simulink model "pfb_fir_real_plan"  (Simulink 7.6)
settings: Solver=ode45  StartTime=0.0  StopTime=10.0  RelTol=1e-3
undefined symbols (not defined in the file or in its folder): pfb_coeff_gen_calc_custom
libraries: xbsIndex_r4 x422, xbsReplacements_r4 x20, monroe_library x15
(part 1 of 4)
settings Model: Creator=monroe  LastModifiedBy=monroe

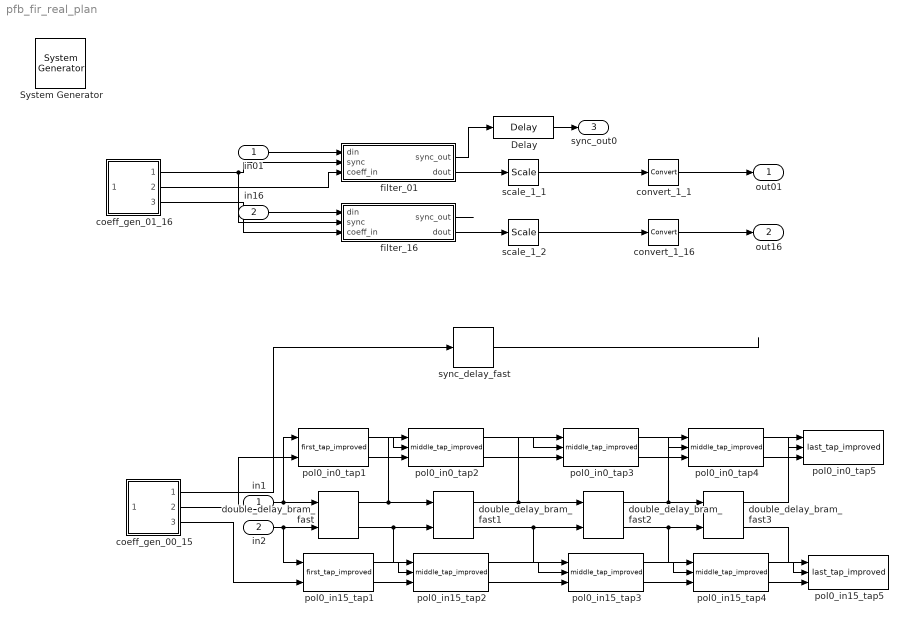
== system pfb_fir_real_plan ==
  in01 : Inport
  in16 : Inport  Port=2
  " System Generator" : xbsIndex_r4/ System Generator  Tag=genX  SystemSampleTime=-1  xilinxfamily=Virtex6  part=xc6vsx315t  speed=-3  package=ff1156  synthesis_tool=XST  clock_wrapper=Clock Enables  directory=./netlist  testbench=off  simulink_period=1  sysclk_period=10  dcm_input_clock_period=10  incr_netlist=off  trim_vbits=Everywhere in SubSystem  dbl_ovrd=According to Block Masks  core_generation=According to Block Masks  run_coregen=off  deprecated_control=off  eval_field=0  block_type=sysgen
  Delay : xbsIndex_r4/Delay  en=off  latency=1  dbl_ovrd=off  reg_retiming=off  block_type=delay
      settings: block_version=11.4
  coeff_gen_00_15 : Subsystem
      settings: AttributesFormatString=PFBSize=14, n_inputs=4, taps=2
  coeff_gen_01_16 : Subsystem
      settings: AttributesFormatString=PFBSize=14, n_inputs=4, taps=2
  convert_1_1 : xbsIndex_r4/Convert  arith_type="Signed  (2's comp)"  n_bits=18  bin_pt=17  quantization=Truncate  overflow=Wrap  en=off  latency=1  dbl_ovrd=off  pipeline=on  block_type=convert
      settings: block_version=11.4
  convert_1_16 : xbsIndex_r4/Convert  arith_type="Signed  (2's comp)"  n_bits=18  bin_pt=17  quantization=Truncate  overflow=Wrap  en=off  latency=1  dbl_ovrd=off  pipeline=on  block_type=convert
      settings: block_version=11.4
  double_delay_bram_fast{,1..3} (4 alike) : monroe_library/double_delay_bram_fast  SystemSampleTime=-1  delay_len=1024  bram_latency=3
  filter_01 : Subsystem
  filter_16 : Subsystem
  in1 : InportShadow  Port=1
  in2 : InportShadow  Port=2
  pol0_in0_tap1 : monroe_library/first_tap_improved  SystemSampleTime=-1  din_bit_width=18  din_bin_pt=17  coeff_bit_width=18  coeff_bin_pt=17
  pol0_in0_tap2 : monroe_library/middle_tap_improved  SystemSampleTime=-1  din_bit_width=18  din_bin_pt=17  coeff_bit_width=18  coeff_bin_pt=17  stage_num=2
  pol0_in0_tap3 : monroe_library/middle_tap_improved  SystemSampleTime=-1  din_bit_width=18  din_bin_pt=17  coeff_bit_width=18  coeff_bin_pt=17  stage_num=2
  pol0_in0_tap4 : monroe_library/middle_tap_improved  SystemSampleTime=-1  din_bit_width=18  din_bin_pt=17  coeff_bit_width=18  coeff_bin_pt=17  stage_num=2
  pol0_in0_tap5 : monroe_library/last_tap_improved  SystemSampleTime=-1  data_bin_pt=17  coeff_bin_pt=17  stage_num=6
  pol0_in15_tap1 : monroe_library/first_tap_improved  SystemSampleTime=-1  din_bit_width=18  din_bin_pt=17  coeff_bit_width=18  coeff_bin_pt=17
  pol0_in15_tap2 : monroe_library/middle_tap_improved  SystemSampleTime=-1  din_bit_width=18  din_bin_pt=17  coeff_bit_width=18  coeff_bin_pt=17  stage_num=2
  pol0_in15_tap3 : monroe_library/middle_tap_improved  SystemSampleTime=-1  din_bit_width=18  din_bin_pt=17  coeff_bit_width=18  coeff_bin_pt=17  stage_num=2
  pol0_in15_tap4 : monroe_library/middle_tap_improved  SystemSampleTime=-1  din_bit_width=18  din_bin_pt=17  coeff_bit_width=18  coeff_bin_pt=17  stage_num=2
  pol0_in15_tap5 : monroe_library/last_tap_improved  SystemSampleTime=-1  data_bin_pt=17  coeff_bin_pt=17  stage_num=6
  scale_1_1 : xbsIndex_r4/Scale  scale_factor=-1  dbl_ovrd=off  block_type=scale
  scale_1_2 : xbsIndex_r4/Scale  scale_factor=-1  dbl_ovrd=off  block_type=scale
  sync_delay_fast : monroe_library/sync_delay_fast  SystemSampleTime=-1  delay_len=1024*5+6+3-1
  out01 : Outport
  out16 : Outport  Port=2
  sync_out0 : Outport  Port=3
  wires:
  filter_16/1(sync_out) -> ?
  filter_16/2(dout) -> scale_1_2/1
  convert_1_16/1 -> out16/1
  scale_1_2/1 -> convert_1_16/1
  filter_01/2(dout) -> scale_1_1/1
  filter_01/1(sync_out) -> Delay/1
  Delay/1 -> sync_out0/1
  convert_1_1/1 -> out01/1
  scale_1_1/1 -> convert_1_1/1
  coeff_gen_01_16/1(sync_out) -> filter_01/2(sync), filter_16/2(sync)
  coeff_gen_01_16/3(coeff_rev) -> filter_16/3(coeff_in)
  coeff_gen_01_16/2(coeff) -> filter_01/3(coeff_in)
  in01/1 -> filter_01/1(din)
  in16/1 -> filter_16/1(din)
  in2/1 -> double_delay_bram_fast/2, pol0_in15_tap1/1
  in1/1 -> double_delay_bram_fast/1, pol0_in0_tap1/1
  double_delay_bram_fast/1 -> double_delay_bram_fast1/1, pol0_in0_tap2/1
  double_delay_bram_fast/2 -> double_delay_bram_fast1/2, pol0_in15_tap2/1
  double_delay_bram_fast1/1 -> double_delay_bram_fast2/1, pol0_in0_tap3/1
  double_delay_bram_fast1/2 -> double_delay_bram_fast2/2, pol0_in15_tap3/1
  double_delay_bram_fast2/1 -> double_delay_bram_fast3/1, pol0_in0_tap4/1
  double_delay_bram_fast2/2 -> double_delay_bram_fast3/2, pol0_in15_tap4/1
  double_delay_bram_fast3/1 -> pol0_in0_tap5/1
  double_delay_bram_fast3/2 -> pol0_in15_tap5/1
  coeff_gen_00_15/1(sync_out) -> sync_delay_fast/1
  sync_delay_fast/1 -> ?
  coeff_gen_00_15/2(coeff) -> pol0_in0_tap1/2
  coeff_gen_00_15/3(coeff_rev) -> pol0_in15_tap1/2
  pol0_in0_tap1/1 -> pol0_in0_tap2/2
  pol0_in0_tap1/2 -> pol0_in0_tap2/3
  pol0_in0_tap2/1 -> pol0_in0_tap3/2
  pol0_in0_tap2/2 -> pol0_in0_tap3/3
  pol0_in0_tap3/1 -> pol0_in0_tap4/2
  pol0_in0_tap3/2 -> pol0_in0_tap4/3
  pol0_in0_tap4/1 -> pol0_in0_tap5/2
  pol0_in0_tap4/2 -> pol0_in0_tap5/3
  pol0_in15_tap1/1 -> pol0_in15_tap2/2
  pol0_in15_tap1/2 -> pol0_in15_tap2/3
  pol0_in15_tap2/1 -> pol0_in15_tap3/2
  pol0_in15_tap2/2 -> pol0_in15_tap3/3
  pol0_in15_tap3/1 -> pol0_in15_tap4/2
  pol0_in15_tap3/2 -> pol0_in15_tap4/3
  pol0_in15_tap4/1 -> pol0_in15_tap5/2
  pol0_in15_tap4/2 -> pol0_in15_tap5/3

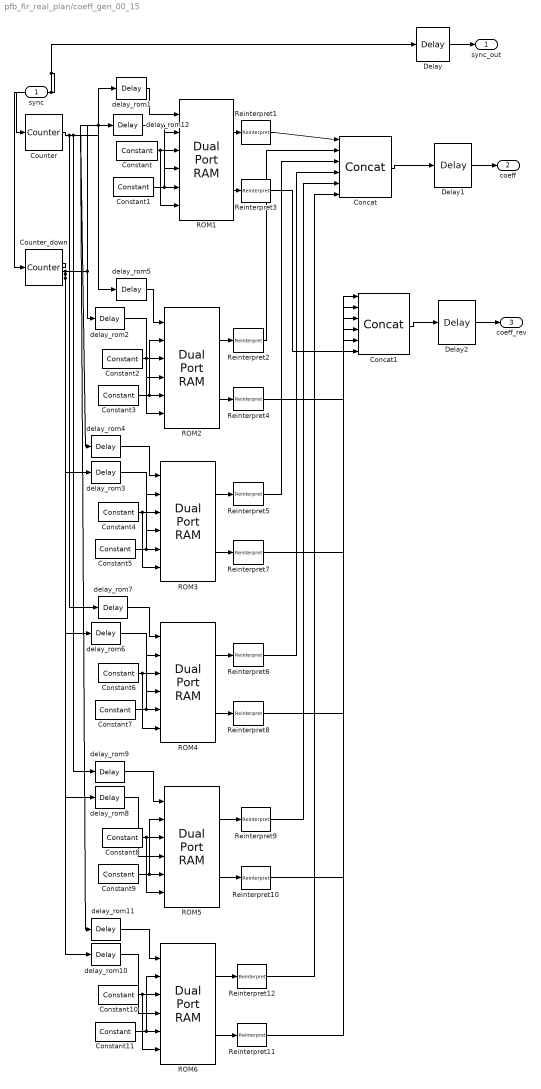
== system pfb_fir_real_plan/coeff_gen_00_15 ==
  sync : Inport
  Concat : xbsIndex_r4/Concat  num_inputs=6  dbl_ovrd=off  block_type=concat
      settings: block_version=9.1.01
  Concat1 : xbsIndex_r4/Concat  num_inputs=6  dbl_ovrd=off  block_type=concat
      settings: block_version=9.1.01
  Constant{,2,4,6,8,10} (6 alike) : xbsIndex_r4/Constant  arith_type=Boolean  const=0  n_bits=16  bin_pt=14  explicit_period=off  period=1  equ=P=C  opselect=C  inp2=PCIN>>17  opr=+  inp1=P  carry=CIN  dbl_ovrd=off  block_type=constant
  Constant{1,3,5,7,9,11} (6 alike) : xbsIndex_r4/Constant  arith_type=Signed (2's comp)  const=0  n_bits=18  bin_pt=17  explicit_period=off  period=1  equ=P=C  opselect=C  inp2=PCIN>>17  opr=+  inp1=P  carry=CIN  dbl_ovrd=off  block_type=constant
  Counter : xbsIndex_r4/Counter  cnt_type=Free Running  cnt_to=Inf  operation=Up  start_count=0  cnt_by_val=1  arith_type=Unsigned  n_bits=10  bin_pt=0  load_pin=off  rst=on  en=off  explicit_period=on  period=1  dbl_ovrd=off  use_behavioral_HDL=off  implementation=Fabric  use_rpm=on  block_type=counter
      settings: xl_area=[0, 0, 0, 0, 0, 0, 0]  block_version=9.1.01
  Counter_down : xbsIndex_r4/Counter  cnt_type=Free Running  cnt_to=Inf  operation=Up  start_count=2^10-1  cnt_by_val=-1  arith_type=Unsigned  n_bits=10  bin_pt=0  load_pin=off  rst=on  en=off  explicit_period=on  period=1  dbl_ovrd=off  use_behavioral_HDL=off  implementation=Fabric  use_rpm=on  block_type=counter
      settings: xl_area=[0, 0, 0, 0, 0, 0, 0]  block_version=9.1.01
  Delay : xbsIndex_r4/Delay  en=off  latency=4  dbl_ovrd=off  reg_retiming=off  block_type=delay
      settings: xl_area=[0, 0, 0, 0, 0, 0, 0]  block_version=9.1.01
  Delay1 : xbsIndex_r4/Delay  en=off  latency=1  dbl_ovrd=off  reg_retiming=off  block_type=delay
  Delay2 : xbsIndex_r4/Delay  en=off  latency=1  dbl_ovrd=off  reg_retiming=off  block_type=delay
  ROM1 : xbsIndex_r4/Dual Port RAM  depth=1024  initVector=pfb_coeff_gen_calc_custom(14,6,4,0,1,1)  distributed_mem=Block RAM  init_a=0  init_b=0  rst_a=off  rst_b=off  en_a=off  en_b=off  latency=3  write_mode_A=No Read On Write  write_mode_B=No Read On Write  dbl_ovrd=off  optimize=Area  use_rpm=on  block_type=dpram
  ROM2 : xbsIndex_r4/Dual Port RAM  depth=1024  initVector=pfb_coeff_gen_calc_custom(14,6,4,0,1,2)  distributed_mem=Block RAM  init_a=0  init_b=0  rst_a=off  rst_b=off  en_a=off  en_b=off  latency=3  write_mode_A=No Read On Write  write_mode_B=No Read On Write  dbl_ovrd=off  optimize=Area  use_rpm=on  block_type=dpram
  ROM3 : xbsIndex_r4/Dual Port RAM  depth=1024  initVector=pfb_coeff_gen_calc_custom(14,6,4,0,1,3)  distributed_mem=Block RAM  init_a=0  init_b=0  rst_a=off  rst_b=off  en_a=off  en_b=off  latency=3  write_mode_A=No Read On Write  write_mode_B=No Read On Write  dbl_ovrd=off  optimize=Area  use_rpm=on  block_type=dpram
  ROM4 : xbsIndex_r4/Dual Port RAM  depth=1024  initVector=pfb_coeff_gen_calc_custom(14,6,4,0,1,4)  distributed_mem=Block RAM  init_a=0  init_b=0  rst_a=off  rst_b=off  en_a=off  en_b=off  latency=3  write_mode_A=No Read On Write  write_mode_B=No Read On Write  dbl_ovrd=off  optimize=Area  use_rpm=on  block_type=dpram
  ROM5 : xbsIndex_r4/Dual Port RAM  depth=1024  initVector=pfb_coeff_gen_calc_custom(14,6,4,0,1,5)  distributed_mem=Block RAM  init_a=0  init_b=0  rst_a=off  rst_b=off  en_a=off  en_b=off  latency=3  write_mode_A=No Read On Write  write_mode_B=No Read On Write  dbl_ovrd=off  optimize=Area  use_rpm=on  block_type=dpram
  ROM6 : xbsIndex_r4/Dual Port RAM  depth=1024  initVector=pfb_coeff_gen_calc_custom(14,6,4,0,1,6)  distributed_mem=Block RAM  init_a=0  init_b=0  rst_a=off  rst_b=off  en_a=off  en_b=off  latency=3  write_mode_A=No Read On Write  write_mode_B=No Read On Write  dbl_ovrd=off  optimize=Area  use_rpm=on  block_type=dpram
  Reinterpret{1..12} (12 alike) : xbsIndex_r4/Reinterpret  force_arith_type=on  arith_type=Unsigned  force_bin_pt=on  bin_pt=0  block_type=reinterpret
      settings: infoedit="Changes signal type without altering the binary representation.   You can changed the signal between signed and unsigned, and relocate the binary point.<P><P>Hardware notes: In hardware this block costs nothing.<P><P>Example:  Suppose the input is 6 bits wide, signed, with 2 fractional bits, and the output is forced to unsigned with 0 fractional bits.  Then an input of -2.0 (1110.00 in binary 2's complement) becomes an output of 56 (111000 in binary)."  block_version=9.1.01
  delay_rom1 : xbsIndex_r4/Delay  en=off  latency=5  dbl_ovrd=off  reg_retiming=off  block_type=delay
  delay_rom10 : xbsIndex_r4/Delay  en=off  latency=5  dbl_ovrd=off  reg_retiming=off  block_type=delay
  delay_rom11 : xbsIndex_r4/Delay  en=off  latency=0  dbl_ovrd=off  reg_retiming=off  block_type=delay
  delay_rom12 : xbsIndex_r4/Delay  en=off  latency=0  dbl_ovrd=off  reg_retiming=off  block_type=delay
  delay_rom2 : xbsIndex_r4/Delay  en=off  latency=1  dbl_ovrd=off  reg_retiming=off  block_type=delay
  delay_rom3 : xbsIndex_r4/Delay  en=off  latency=2  dbl_ovrd=off  reg_retiming=off  block_type=delay
  delay_rom4 : xbsIndex_r4/Delay  en=off  latency=3  dbl_ovrd=off  reg_retiming=off  block_type=delay
  delay_rom5 : xbsIndex_r4/Delay  en=off  latency=4  dbl_ovrd=off  reg_retiming=off  block_type=delay
  delay_rom6 : xbsIndex_r4/Delay  en=off  latency=3  dbl_ovrd=off  reg_retiming=off  block_type=delay
  delay_rom7 : xbsIndex_r4/Delay  en=off  latency=2  dbl_ovrd=off  reg_retiming=off  block_type=delay
  delay_rom8 : xbsIndex_r4/Delay  en=off  latency=4  dbl_ovrd=off  reg_retiming=off  block_type=delay
  delay_rom9 : xbsIndex_r4/Delay  en=off  latency=1  dbl_ovrd=off  reg_retiming=off  block_type=delay
  sync_out : Outport
  coeff : Outport  Port=2
  coeff_rev : Outport  Port=3
  wires:
  Concat1/1 -> Delay2/1
  Delay2/1 -> coeff_rev/1
  Counter_down/1 -> delay_rom2/1, delay_rom12/1, delay_rom3/1, delay_rom6/1, delay_rom8/1, delay_rom10/1
  ROM1/2 -> Reinterpret3/1
  ROM2/1 -> Reinterpret2/1
  Constant3/1 -> ROM2/5, ROM2/2
  Constant2/1 -> ROM2/3, ROM2/6
  Constant1/1 -> ROM1/2, ROM1/5
  Constant/1 -> ROM1/6, ROM1/3
  Reinterpret2/1 -> Concat/2
  Reinterpret1/1 -> Concat/1
  ROM1/1 -> Reinterpret1/1
  Counter/1 -> delay_rom7/1, delay_rom1/1, delay_rom5/1, delay_rom4/1, delay_rom11/1, delay_rom9/1
  Delay1/1 -> coeff/1
  Concat/1 -> Delay1/1
  Delay/1 -> sync_out/1
  sync/1 -> Counter_down/1, Delay/1, Counter/1
  ROM2/2 -> Reinterpret4/1
  delay_rom1/1 -> ROM1/1
  delay_rom2/1 -> ROM2/4
  Constant5/1 -> ROM3/2, ROM3/5
  Constant4/1 -> ROM3/6, ROM3/3
  delay_rom3/1 -> ROM3/4
  delay_rom5/1 -> ROM2/1
  delay_rom4/1 -> ROM3/1
  Constant7/1 -> ROM4/5, ROM4/2
  Constant6/1 -> ROM4/3, ROM4/6
  delay_rom6/1 -> ROM4/4
  delay_rom7/1 -> ROM4/1
  Constant9/1 -> ROM5/2, ROM5/5
  Constant8/1 -> ROM5/6, ROM5/3
  delay_rom8/1 -> ROM5/4
  delay_rom9/1 -> ROM5/1
  Constant11/1 -> ROM6/5, ROM6/2
  Constant10/1 -> ROM6/3, ROM6/6
  delay_rom10/1 -> ROM6/4
  delay_rom11/1 -> ROM6/1
  Reinterpret3/1 -> Concat1/6
  Reinterpret4/1 -> Concat1/5
  ROM3/1 -> Reinterpret5/1
  ROM3/2 -> Reinterpret7/1
  ROM4/1 -> Reinterpret6/1
  ROM4/2 -> Reinterpret8/1
  ROM5/1 -> Reinterpret9/1
  ROM5/2 -> Reinterpret10/1
  ROM6/1 -> Reinterpret12/1
  ROM6/2 -> Reinterpret11/1
  Reinterpret5/1 -> Concat/3
  Reinterpret6/1 -> Concat/4
  Reinterpret9/1 -> Concat/5
  Reinterpret12/1 -> Concat/6
  Reinterpret7/1 -> Concat1/4
  Reinterpret8/1 -> Concat1/3
  Reinterpret10/1 -> Concat1/2
  Reinterpret11/1 -> Concat1/1
  delay_rom12/1 -> ROM1/4

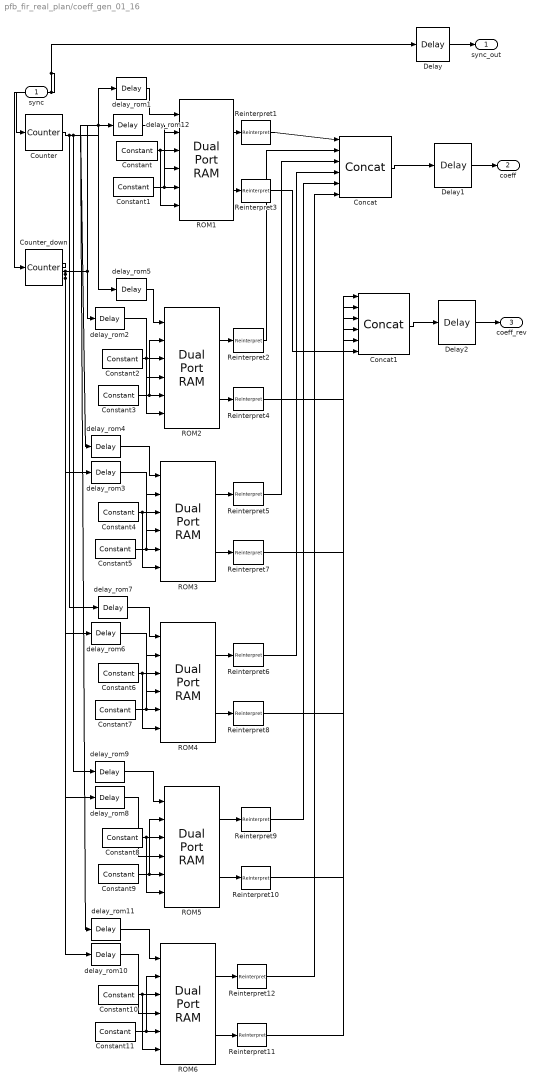
== system pfb_fir_real_plan/coeff_gen_01_16 ==
  sync : Inport
  Concat : xbsIndex_r4/Concat  num_inputs=6  dbl_ovrd=off  block_type=concat
      settings: block_version=9.1.01
  Concat1 : xbsIndex_r4/Concat  num_inputs=6  dbl_ovrd=off  block_type=concat
      settings: block_version=9.1.01
  Constant{,2,4,6,8,10} (6 alike) : xbsIndex_r4/Constant  arith_type=Boolean  const=0  n_bits=16  bin_pt=14  explicit_period=off  period=1  equ=P=C  opselect=C  inp2=PCIN>>17  opr=+  inp1=P  carry=CIN  dbl_ovrd=off  block_type=constant
  Constant{1,3,5,7,9,11} (6 alike) : xbsIndex_r4/Constant  arith_type=Signed (2's comp)  const=0  n_bits=18  bin_pt=17  explicit_period=off  period=1  equ=P=C  opselect=C  inp2=PCIN>>17  opr=+  inp1=P  carry=CIN  dbl_ovrd=off  block_type=constant
  Counter : xbsIndex_r4/Counter  cnt_type=Free Running  cnt_to=Inf  operation=Up  start_count=0  cnt_by_val=1  arith_type=Unsigned  n_bits=10  bin_pt=0  load_pin=off  rst=on  en=off  explicit_period=on  period=1  dbl_ovrd=off  use_behavioral_HDL=off  implementation=Fabric  use_rpm=on  block_type=counter
      settings: xl_area=[0, 0, 0, 0, 0, 0, 0]  block_version=9.1.01
  Counter_down : xbsIndex_r4/Counter  cnt_type=Free Running  cnt_to=Inf  operation=Up  start_count=2^10-1  cnt_by_val=-1  arith_type=Unsigned  n_bits=10  bin_pt=0  load_pin=off  rst=on  en=off  explicit_period=on  period=1  dbl_ovrd=off  use_behavioral_HDL=off  implementation=Fabric  use_rpm=on  block_type=counter
      settings: xl_area=[0, 0, 0, 0, 0, 0, 0]  block_version=9.1.01
  Delay : xbsIndex_r4/Delay  en=off  latency=4  dbl_ovrd=off  reg_retiming=off  block_type=delay
      settings: xl_area=[0, 0, 0, 0, 0, 0, 0]  block_version=9.1.01
  Delay1 : xbsIndex_r4/Delay  en=off  latency=1  dbl_ovrd=off  reg_retiming=off  block_type=delay
  Delay2 : xbsIndex_r4/Delay  en=off  latency=1  dbl_ovrd=off  reg_retiming=off  block_type=delay
  ROM1 : xbsIndex_r4/Dual Port RAM  depth=1024  initVector=pfb_coeff_gen_calc_custom(14,6,4,0,1,1)  distributed_mem=Block RAM  init_a=0  init_b=0  rst_a=off  rst_b=off  en_a=off  en_b=off  latency=3  write_mode_A=No Read On Write  write_mode_B=No Read On Write  dbl_ovrd=off  optimize=Area  use_rpm=on  block_type=dpram
  ROM2 : xbsIndex_r4/Dual Port RAM  depth=1024  initVector=pfb_coeff_gen_calc_custom(14,6,4,0,1,2)  distributed_mem=Block RAM  init_a=0  init_b=0  rst_a=off  rst_b=off  en_a=off  en_b=off  latency=3  write_mode_A=No Read On Write  write_mode_B=No Read On Write  dbl_ovrd=off  optimize=Area  use_rpm=on  block_type=dpram
  ROM3 : xbsIndex_r4/Dual Port RAM  depth=1024  initVector=pfb_coeff_gen_calc_custom(14,6,4,0,1,3)  distributed_mem=Block RAM  init_a=0  init_b=0  rst_a=off  rst_b=off  en_a=off  en_b=off  latency=3  write_mode_A=No Read On Write  write_mode_B=No Read On Write  dbl_ovrd=off  optimize=Area  use_rpm=on  block_type=dpram
  ROM4 : xbsIndex_r4/Dual Port RAM  depth=1024  initVector=pfb_coeff_gen_calc_custom(14,6,4,0,1,4)  distributed_mem=Block RAM  init_a=0  init_b=0  rst_a=off  rst_b=off  en_a=off  en_b=off  latency=3  write_mode_A=No Read On Write  write_mode_B=No Read On Write  dbl_ovrd=off  optimize=Area  use_rpm=on  block_type=dpram
  ROM5 : xbsIndex_r4/Dual Port RAM  depth=1024  initVector=pfb_coeff_gen_calc_custom(14,6,4,0,1,5)  distributed_mem=Block RAM  init_a=0  init_b=0  rst_a=off  rst_b=off  en_a=off  en_b=off  latency=3  write_mode_A=No Read On Write  write_mode_B=No Read On Write  dbl_ovrd=off  optimize=Area  use_rpm=on  block_type=dpram
  ROM6 : xbsIndex_r4/Dual Port RAM  depth=1024  initVector=pfb_coeff_gen_calc_custom(14,6,4,0,1,6)  distributed_mem=Block RAM  init_a=0  init_b=0  rst_a=off  rst_b=off  en_a=off  en_b=off  latency=3  write_mode_A=No Read On Write  write_mode_B=No Read On Write  dbl_ovrd=off  optimize=Area  use_rpm=on  block_type=dpram
  Reinterpret{1..12} (12 alike) : xbsIndex_r4/Reinterpret  force_arith_type=on  arith_type=Unsigned  force_bin_pt=on  bin_pt=0  block_type=reinterpret
      settings: infoedit="Changes signal type without altering the binary representation.   You can changed the signal between signed and unsigned, and relocate the binary point.<P><P>Hardware notes: In hardware this block costs nothing.<P><P>Example:  Suppose the input is 6 bits wide, signed, with 2 fractional bits, and the output is forced to unsigned with 0 fractional bits.  Then an input of -2.0 (1110.00 in binary 2's complement) becomes an output of 56 (111000 in binary)."  block_version=9.1.01
  delay_rom1 : xbsIndex_r4/Delay  en=off  latency=5  dbl_ovrd=off  reg_retiming=off  block_type=delay
  delay_rom10 : xbsIndex_r4/Delay  en=off  latency=5  dbl_ovrd=off  reg_retiming=off  block_type=delay
  delay_rom11 : xbsIndex_r4/Delay  en=off  latency=0  dbl_ovrd=off  reg_retiming=off  block_type=delay
  delay_rom12 : xbsIndex_r4/Delay  en=off  latency=0  dbl_ovrd=off  reg_retiming=off  block_type=delay
  delay_rom2 : xbsIndex_r4/Delay  en=off  latency=1  dbl_ovrd=off  reg_retiming=off  block_type=delay
  delay_rom3 : xbsIndex_r4/Delay  en=off  latency=2  dbl_ovrd=off  reg_retiming=off  block_type=delay
  delay_rom4 : xbsIndex_r4/Delay  en=off  latency=3  dbl_ovrd=off  reg_retiming=off  block_type=delay
  delay_rom5 : xbsIndex_r4/Delay  en=off  latency=4  dbl_ovrd=off  reg_retiming=off  block_type=delay
  delay_rom6 : xbsIndex_r4/Delay  en=off  latency=3  dbl_ovrd=off  reg_retiming=off  block_type=delay
  delay_rom7 : xbsIndex_r4/Delay  en=off  latency=2  dbl_ovrd=off  reg_retiming=off  block_type=delay
  delay_rom8 : xbsIndex_r4/Delay  en=off  latency=4  dbl_ovrd=off  reg_retiming=off  block_type=delay
  delay_rom9 : xbsIndex_r4/Delay  en=off  latency=1  dbl_ovrd=off  reg_retiming=off  block_type=delay
  sync_out : Outport
  coeff : Outport  Port=2
  coeff_rev : Outport  Port=3
  wires:
  delay_rom12/1 -> ROM1/4
  Reinterpret11/1 -> Concat1/1
  Reinterpret10/1 -> Concat1/2
  Reinterpret8/1 -> Concat1/3
  Reinterpret7/1 -> Concat1/4
  Reinterpret12/1 -> Concat/6
  Reinterpret9/1 -> Concat/5
  Reinterpret6/1 -> Concat/4
  Reinterpret5/1 -> Concat/3
  ROM6/2 -> Reinterpret11/1
  ROM6/1 -> Reinterpret12/1
  ROM5/2 -> Reinterpret10/1
  ROM5/1 -> Reinterpret9/1
  ROM4/2 -> Reinterpret8/1
  ROM4/1 -> Reinterpret6/1
  ROM3/2 -> Reinterpret7/1
  ROM3/1 -> Reinterpret5/1
  Reinterpret4/1 -> Concat1/5
  Reinterpret3/1 -> Concat1/6
  delay_rom11/1 -> ROM6/1
  delay_rom10/1 -> ROM6/4
  Constant10/1 -> ROM6/6, ROM6/3
  Constant11/1 -> ROM6/2, ROM6/5
  delay_rom9/1 -> ROM5/1
  delay_rom8/1 -> ROM5/4
  Constant8/1 -> ROM5/3, ROM5/6
  Constant9/1 -> ROM5/5, ROM5/2
  delay_rom7/1 -> ROM4/1
  delay_rom6/1 -> ROM4/4
  Constant6/1 -> ROM4/6, ROM4/3
  Constant7/1 -> ROM4/2, ROM4/5
  delay_rom4/1 -> ROM3/1
  delay_rom5/1 -> ROM2/1
  delay_rom3/1 -> ROM3/4
  Constant4/1 -> ROM3/3, ROM3/6
  Constant5/1 -> ROM3/5, ROM3/2
  delay_rom2/1 -> ROM2/4
  delay_rom1/1 -> ROM1/1
  ROM2/2 -> Reinterpret4/1
  sync/1 -> Counter/1, Delay/1, Counter_down/1
  Delay/1 -> sync_out/1
  Concat/1 -> Delay1/1
  Delay1/1 -> coeff/1
  Counter/1 -> delay_rom9/1, delay_rom11/1, delay_rom4/1, delay_rom5/1, delay_rom1/1, delay_rom7/1
  ROM1/1 -> Reinterpret1/1
  Reinterpret1/1 -> Concat/1
  Reinterpret2/1 -> Concat/2
  Constant/1 -> ROM1/3, ROM1/6
  Constant1/1 -> ROM1/5, ROM1/2
  Constant2/1 -> ROM2/6, ROM2/3
  Constant3/1 -> ROM2/2, ROM2/5
  ROM2/1 -> Reinterpret2/1
  ROM1/2 -> Reinterpret3/1
  Counter_down/1 -> delay_rom10/1, delay_rom8/1, delay_rom6/1, delay_rom3/1, delay_rom12/1, delay_rom2/1
  Delay2/1 -> coeff_rev/1
  Concat1/1 -> Delay2/1

== system pfb_fir_real_plan/filter_01 ==
  din : Inport
  sync : Inport  Port=2
  coeff_in : Inport  Port=3
  Delay1 : xbsIndex_r4/Delay  en=off  latency=1  dbl_ovrd=off  reg_retiming=off  block_type=delay
      settings: xl_area=[0, 0, 0, 0, 0, 0, 0]  block_version=9.1.01
  Reinterpret2 : xbsIndex_r4/Reinterpret  force_arith_type=on  arith_type="Signed  (2's comp)"  force_bin_pt=on  bin_pt=34  block_type=reinterpret
      settings: infoedit="Changes signal type without altering the binary representation.   You can changed the signal between signed and unsigned, and relocate the binary point.<br><br>Hardware notes: In hardware this block costs nothing.<br><br>Example:  Suppose the input is 6 bits wide, signed, with 2 fractional bits, and the output is forced to unsigned with 0 fractional bits.  Then an input of -2.0 (1110.00 in binary 2's complement) becomes an output of 56 (111000 in binary)."  block_version=11.3
  tap1 : Subsystem  AncestorBlock=casper_library/PFBs/tap_real
  tap2 : Subsystem  AncestorBlock=casper_library/PFBs/tap_real
  tap3 : Subsystem  AncestorBlock=casper_library/PFBs/tap_real
  tap4 : Subsystem  AncestorBlock=casper_library/PFBs/tap_real
  tap5 : Subsystem  AncestorBlock=casper_library/PFBs/tap_real
  tap6 : Subsystem  AncestorBlock=casper_library/PFBs/last_tap_real
  sync_out : Outport
  dout : Outport  Port=2
  wires:
  tap5/1(dout) -> tap6/1(din)
  tap5/2(sync_out) -> tap6/2(sync)
  tap5/3(coeff_out) -> tap6/3(coeff)
  tap5/4(taps_out) -> tap6/4(tap_in)
  tap1/1(dout) -> tap2/1(din)
  tap1/2(sync_out) -> tap2/2(sync)
  tap1/3(coeff_out) -> tap2/3(coeff)
  tap1/4(taps_out) -> tap2/4(tap_in)
  tap2/1(dout) -> tap3/1(din)
  tap2/2(sync_out) -> tap3/2(sync)
  tap2/3(coeff_out) -> tap3/3(coeff)
  tap2/4(taps_out) -> tap3/4(tap_in)
  tap3/1(dout) -> tap4/1(din)
  tap3/2(sync_out) -> tap4/2(sync)
  tap3/3(coeff_out) -> tap4/3(coeff)
  tap3/4(taps_out) -> tap4/4(tap_in)
  tap4/1(dout) -> tap5/1(din)
  tap4/2(sync_out) -> tap5/2(sync)
  tap4/3(coeff_out) -> tap5/3(coeff)
  tap4/4(taps_out) -> tap5/4(tap_in)
  tap6/2(tap_out) -> Reinterpret2/1
  Delay1/1 -> tap1/1(din)
  din/1 -> Delay1/1
  tap6/1(sync_out) -> sync_out/1
  sync/1 -> tap1/2(sync)
  Reinterpret2/1 -> dout/1
  coeff_in/1 -> tap1/3(coeff)

== system pfb_fir_real_plan/filter_16 ==
  din : Inport
  sync : Inport  Port=2
  coeff_in : Inport  Port=3
  Delay1 : xbsIndex_r4/Delay  en=off  latency=1  dbl_ovrd=off  reg_retiming=off  block_type=delay
      settings: xl_area=[0, 0, 0, 0, 0, 0, 0]  block_version=9.1.01
  Reinterpret2 : xbsIndex_r4/Reinterpret  force_arith_type=on  arith_type="Signed  (2's comp)"  force_bin_pt=on  bin_pt=34  block_type=reinterpret
      settings: infoedit="Changes signal type without altering the binary representation.   You can changed the signal between signed and unsigned, and relocate the binary point.<br><br>Hardware notes: In hardware this block costs nothing.<br><br>Example:  Suppose the input is 6 bits wide, signed, with 2 fractional bits, and the output is forced to unsigned with 0 fractional bits.  Then an input of -2.0 (1110.00 in binary 2's complement) becomes an output of 56 (111000 in binary)."  block_version=11.3
  tap1 : Subsystem  AncestorBlock=casper_library/PFBs/tap_real
  tap2 : Subsystem  AncestorBlock=casper_library/PFBs/tap_real
  tap3 : Subsystem  AncestorBlock=casper_library/PFBs/tap_real
  tap4 : Subsystem  AncestorBlock=casper_library/PFBs/tap_real
  tap5 : Subsystem  AncestorBlock=casper_library/PFBs/tap_real
  tap6 : Subsystem  AncestorBlock=casper_library/PFBs/last_tap_real
  sync_out : Outport
  dout : Outport  Port=2
  wires:
  coeff_in/1 -> tap1/3(coeff)
  Reinterpret2/1 -> dout/1
  sync/1 -> tap1/2(sync)
  tap6/1(sync_out) -> sync_out/1
  din/1 -> Delay1/1
  Delay1/1 -> tap1/1(din)
  tap6/2(tap_out) -> Reinterpret2/1
  tap4/4(taps_out) -> tap5/4(tap_in)
  tap4/3(coeff_out) -> tap5/3(coeff)
  tap4/2(sync_out) -> tap5/2(sync)
  tap4/1(dout) -> tap5/1(din)
  tap3/4(taps_out) -> tap4/4(tap_in)
  tap3/3(coeff_out) -> tap4/3(coeff)
  tap3/2(sync_out) -> tap4/2(sync)
  tap3/1(dout) -> tap4/1(din)
  tap2/4(taps_out) -> tap3/4(tap_in)
  tap2/3(coeff_out) -> tap3/3(coeff)
  tap2/2(sync_out) -> tap3/2(sync)
  tap2/1(dout) -> tap3/1(din)
  tap1/4(taps_out) -> tap2/4(tap_in)
  tap1/3(coeff_out) -> tap2/3(coeff)
  tap1/2(sync_out) -> tap2/2(sync)
  tap1/1(dout) -> tap2/1(din)
  tap5/4(taps_out) -> tap6/4(tap_in)
  tap5/3(coeff_out) -> tap6/3(coeff)
  tap5/2(sync_out) -> tap6/2(sync)
  tap5/1(dout) -> tap6/1(din)

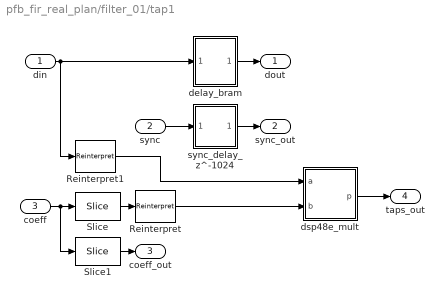
== system pfb_fir_real_plan/filter_01/tap1 ==
  din : Inport
  sync : Inport  Port=2
  coeff : Inport  Port=3
  Reinterpret : xbsIndex_r4/Reinterpret  force_arith_type=on  arith_type="Signed  (2's comp)"  force_bin_pt=on  bin_pt=17  block_type=reinterpret
      settings: infoedit="Changes signal type without altering the binary representation.   You can changed the signal between signed and unsigned, and relocate the binary point.<br><br>Hardware notes: In hardware this block costs nothing.<br><br>Example:  Suppose the input is 6 bits wide, signed, with 2 fractional bits, and the output is forced to unsigned with 0 fractional bits.  Then an input of -2.0 (1110.00 in binary 2's complement) becomes an output of 56 (111000 in binary)."  block_version=9.1.01
  Reinterpret1 : xbsIndex_r4/Reinterpret  force_arith_type=on  arith_type="Signed  (2's comp)"  force_bin_pt=on  bin_pt=17  block_type=reinterpret
      settings: infoedit="Changes signal type without altering the binary representation.   You can changed the signal between signed and unsigned, and relocate the binary point.<br><br>Hardware notes: In hardware this block costs nothing.<br><br>Example:  Suppose the input is 6 bits wide, signed, with 2 fractional bits, and the output is forced to unsigned with 0 fractional bits.  Then an input of -2.0 (1110.00 in binary 2's complement) becomes an output of 56 (111000 in binary)."  block_version=9.1.01
  Slice : xbsIndex_r4/Slice  nbits=18  boolean_output=off  mode=Lower Bit Location + Width  bit1=0  base1=MSB of Input  bit0=0  base0=LSB of Input  dbl_ovrd=off  block_type=slice
      settings: block_version=9.1.01
  Slice1 : xbsIndex_r4/Slice  nbits=0  boolean_output=off  mode=Two Bit Locations  bit1=0  base1=MSB of Input  bit0=18  base0=LSB of Input  dbl_ovrd=off  block_type=slice
      settings: block_version=9.1.01
  delay_bram : Subsystem
  dsp48e_mult : Subsystem
  sync_delay_z^-1024 : Subsystem
  dout : Outport
  sync_out : Outport  Port=2
  coeff_out : Outport  Port=3
  taps_out : Outport  Port=4
  wires:
  Reinterpret1/1 -> dsp48e_mult/1(a)
  Reinterpret/1 -> dsp48e_mult/2(b)
  Slice/1 -> Reinterpret/1
  Slice1/1 -> coeff_out/1
  coeff/1 -> Slice1/1, Slice/1
  sync_delay_z^-1024/1(Out1) -> sync_out/1
  sync/1 -> sync_delay_z^-1024/1(In1)
  dsp48e_mult/1(p) -> taps_out/1
  din/1 -> Reinterpret1/1, delay_bram/1(In1)
  delay_bram/1(Out1) -> dout/1

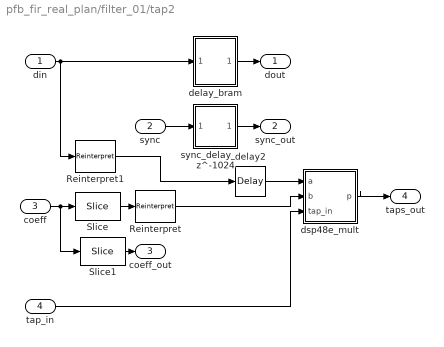
== system pfb_fir_real_plan/filter_01/tap2 ==
  din : Inport
  sync : Inport  Port=2
  coeff : Inport  Port=3
  tap_in : Inport  Port=4
  Reinterpret : xbsIndex_r4/Reinterpret  force_arith_type=on  arith_type="Signed  (2's comp)"  force_bin_pt=on  bin_pt=17  block_type=reinterpret
      settings: infoedit="Changes signal type without altering the binary representation.   You can changed the signal between signed and unsigned, and relocate the binary point.<br><br>Hardware notes: In hardware this block costs nothing.<br><br>Example:  Suppose the input is 6 bits wide, signed, with 2 fractional bits, and the output is forced to unsigned with 0 fractional bits.  Then an input of -2.0 (1110.00 in binary 2's complement) becomes an output of 56 (111000 in binary)."  block_version=9.1.01
  Reinterpret1 : xbsIndex_r4/Reinterpret  force_arith_type=on  arith_type="Signed  (2's comp)"  force_bin_pt=on  bin_pt=17  block_type=reinterpret
      settings: infoedit="Changes signal type without altering the binary representation.   You can changed the signal between signed and unsigned, and relocate the binary point.<br><br>Hardware notes: In hardware this block costs nothing.<br><br>Example:  Suppose the input is 6 bits wide, signed, with 2 fractional bits, and the output is forced to unsigned with 0 fractional bits.  Then an input of -2.0 (1110.00 in binary 2's complement) becomes an output of 56 (111000 in binary)."  block_version=9.1.01
  Slice : xbsIndex_r4/Slice  nbits=18  boolean_output=off  mode=Lower Bit Location + Width  bit1=0  base1=MSB of Input  bit0=0  base0=LSB of Input  dbl_ovrd=off  block_type=slice
      settings: block_version=9.1.01
  Slice1 : xbsIndex_r4/Slice  nbits=0  boolean_output=off  mode=Two Bit Locations  bit1=0  base1=MSB of Input  bit0=18  base0=LSB of Input  dbl_ovrd=off  block_type=slice
      settings: block_version=9.1.01
  delay2 : xbsIndex_r4/Delay  en=off  latency=1  dbl_ovrd=off  reg_retiming=off  block_type=delay
  delay_bram : Subsystem
  dsp48e_mult : Subsystem
  sync_delay_z^-1024 : Subsystem
  dout : Outport
  sync_out : Outport  Port=2
  coeff_out : Outport  Port=3
  taps_out : Outport  Port=4
  wires:
  delay_bram/1(Out1) -> dout/1
  din/1 -> delay_bram/1(In1), Reinterpret1/1
  dsp48e_mult/1(p) -> taps_out/1
  sync/1 -> sync_delay_z^-1024/1(In1)
  sync_delay_z^-1024/1(Out1) -> sync_out/1
  coeff/1 -> Slice/1, Slice1/1
  Slice1/1 -> coeff_out/1
  Slice/1 -> Reinterpret/1
  Reinterpret/1 -> dsp48e_mult/2(b)
  delay2/1 -> dsp48e_mult/1(a)
  Reinterpret1/1 -> delay2/1
  tap_in/1 -> dsp48e_mult/3(tap_in)

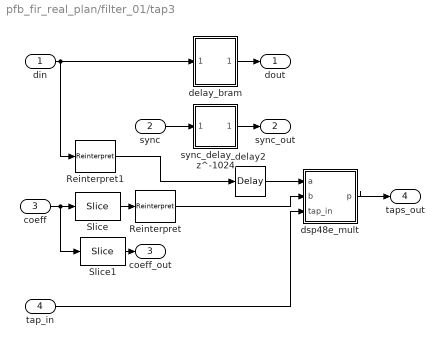
== system pfb_fir_real_plan/filter_01/tap3 ==
  din : Inport
  sync : Inport  Port=2
  coeff : Inport  Port=3
  tap_in : Inport  Port=4
  Reinterpret : xbsIndex_r4/Reinterpret  force_arith_type=on  arith_type="Signed  (2's comp)"  force_bin_pt=on  bin_pt=17  block_type=reinterpret
      settings: infoedit="Changes signal type without altering the binary representation.   You can changed the signal between signed and unsigned, and relocate the binary point.<br><br>Hardware notes: In hardware this block costs nothing.<br><br>Example:  Suppose the input is 6 bits wide, signed, with 2 fractional bits, and the output is forced to unsigned with 0 fractional bits.  Then an input of -2.0 (1110.00 in binary 2's complement) becomes an output of 56 (111000 in binary)."  block_version=9.1.01
  Reinterpret1 : xbsIndex_r4/Reinterpret  force_arith_type=on  arith_type="Signed  (2's comp)"  force_bin_pt=on  bin_pt=17  block_type=reinterpret
      settings: infoedit="Changes signal type without altering the binary representation.   You can changed the signal between signed and unsigned, and relocate the binary point.<br><br>Hardware notes: In hardware this block costs nothing.<br><br>Example:  Suppose the input is 6 bits wide, signed, with 2 fractional bits, and the output is forced to unsigned with 0 fractional bits.  Then an input of -2.0 (1110.00 in binary 2's complement) becomes an output of 56 (111000 in binary)."  block_version=9.1.01
  Slice : xbsIndex_r4/Slice  nbits=18  boolean_output=off  mode=Lower Bit Location + Width  bit1=0  base1=MSB of Input  bit0=0  base0=LSB of Input  dbl_ovrd=off  block_type=slice
      settings: block_version=9.1.01
  Slice1 : xbsIndex_r4/Slice  nbits=0  boolean_output=off  mode=Two Bit Locations  bit1=0  base1=MSB of Input  bit0=18  base0=LSB of Input  dbl_ovrd=off  block_type=slice
      settings: block_version=9.1.01
  delay2 : xbsIndex_r4/Delay  en=off  latency=2  dbl_ovrd=off  reg_retiming=off  block_type=delay
  delay_bram : Subsystem
  dsp48e_mult : Subsystem
  sync_delay_z^-1024 : Subsystem
  dout : Outport
  sync_out : Outport  Port=2
  coeff_out : Outport  Port=3
  taps_out : Outport  Port=4
  wires:
  tap_in/1 -> dsp48e_mult/3(tap_in)
  Reinterpret1/1 -> delay2/1
  delay2/1 -> dsp48e_mult/1(a)
  Reinterpret/1 -> dsp48e_mult/2(b)
  Slice/1 -> Reinterpret/1
  Slice1/1 -> coeff_out/1
  coeff/1 -> Slice1/1, Slice/1
  sync_delay_z^-1024/1(Out1) -> sync_out/1
  sync/1 -> sync_delay_z^-1024/1(In1)
  dsp48e_mult/1(p) -> taps_out/1
  din/1 -> Reinterpret1/1, delay_bram/1(In1)
  delay_bram/1(Out1) -> dout/1

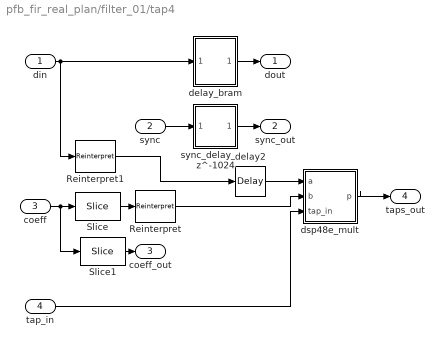
== system pfb_fir_real_plan/filter_01/tap4 ==
  din : Inport
  sync : Inport  Port=2
  coeff : Inport  Port=3
  tap_in : Inport  Port=4
  Reinterpret : xbsIndex_r4/Reinterpret  force_arith_type=on  arith_type="Signed  (2's comp)"  force_bin_pt=on  bin_pt=17  block_type=reinterpret
      settings: infoedit="Changes signal type without altering the binary representation.   You can changed the signal between signed and unsigned, and relocate the binary point.<br><br>Hardware notes: In hardware this block costs nothing.<br><br>Example:  Suppose the input is 6 bits wide, signed, with 2 fractional bits, and the output is forced to unsigned with 0 fractional bits.  Then an input of -2.0 (1110.00 in binary 2's complement) becomes an output of 56 (111000 in binary)."  block_version=9.1.01
  Reinterpret1 : xbsIndex_r4/Reinterpret  force_arith_type=on  arith_type="Signed  (2's comp)"  force_bin_pt=on  bin_pt=17  block_type=reinterpret
      settings: infoedit="Changes signal type without altering the binary representation.   You can changed the signal between signed and unsigned, and relocate the binary point.<br><br>Hardware notes: In hardware this block costs nothing.<br><br>Example:  Suppose the input is 6 bits wide, signed, with 2 fractional bits, and the output is forced to unsigned with 0 fractional bits.  Then an input of -2.0 (1110.00 in binary 2's complement) becomes an output of 56 (111000 in binary)."  block_version=9.1.01
  Slice : xbsIndex_r4/Slice  nbits=18  boolean_output=off  mode=Lower Bit Location + Width  bit1=0  base1=MSB of Input  bit0=0  base0=LSB of Input  dbl_ovrd=off  block_type=slice
      settings: block_version=9.1.01
  Slice1 : xbsIndex_r4/Slice  nbits=0  boolean_output=off  mode=Two Bit Locations  bit1=0  base1=MSB of Input  bit0=18  base0=LSB of Input  dbl_ovrd=off  block_type=slice
      settings: block_version=9.1.01
  delay2 : xbsIndex_r4/Delay  en=off  latency=3  dbl_ovrd=off  reg_retiming=off  block_type=delay
  delay_bram : Subsystem
  dsp48e_mult : Subsystem
  sync_delay_z^-1024 : Subsystem
  dout : Outport
  sync_out : Outport  Port=2
  coeff_out : Outport  Port=3
  taps_out : Outport  Port=4
  wires:
  delay_bram/1(Out1) -> dout/1
  din/1 -> delay_bram/1(In1), Reinterpret1/1
  dsp48e_mult/1(p) -> taps_out/1
  sync/1 -> sync_delay_z^-1024/1(In1)
  sync_delay_z^-1024/1(Out1) -> sync_out/1
  coeff/1 -> Slice/1, Slice1/1
  Slice1/1 -> coeff_out/1
  Slice/1 -> Reinterpret/1
  Reinterpret/1 -> dsp48e_mult/2(b)
  delay2/1 -> dsp48e_mult/1(a)
  Reinterpret1/1 -> delay2/1
  tap_in/1 -> dsp48e_mult/3(tap_in)

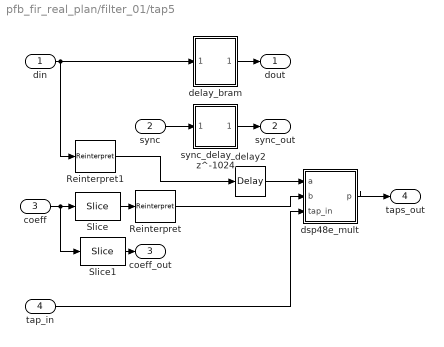
== system pfb_fir_real_plan/filter_01/tap5 ==
  din : Inport
  sync : Inport  Port=2
  coeff : Inport  Port=3
  tap_in : Inport  Port=4
  Reinterpret : xbsIndex_r4/Reinterpret  force_arith_type=on  arith_type="Signed  (2's comp)"  force_bin_pt=on  bin_pt=17  block_type=reinterpret
      settings: infoedit="Changes signal type without altering the binary representation.   You can changed the signal between signed and unsigned, and relocate the binary point.<br><br>Hardware notes: In hardware this block costs nothing.<br><br>Example:  Suppose the input is 6 bits wide, signed, with 2 fractional bits, and the output is forced to unsigned with 0 fractional bits.  Then an input of -2.0 (1110.00 in binary 2's complement) becomes an output of 56 (111000 in binary)."  block_version=9.1.01
  Reinterpret1 : xbsIndex_r4/Reinterpret  force_arith_type=on  arith_type="Signed  (2's comp)"  force_bin_pt=on  bin_pt=17  block_type=reinterpret
      settings: infoedit="Changes signal type without altering the binary representation.   You can changed the signal between signed and unsigned, and relocate the binary point.<br><br>Hardware notes: In hardware this block costs nothing.<br><br>Example:  Suppose the input is 6 bits wide, signed, with 2 fractional bits, and the output is forced to unsigned with 0 fractional bits.  Then an input of -2.0 (1110.00 in binary 2's complement) becomes an output of 56 (111000 in binary)."  block_version=9.1.01
  Slice : xbsIndex_r4/Slice  nbits=18  boolean_output=off  mode=Lower Bit Location + Width  bit1=0  base1=MSB of Input  bit0=0  base0=LSB of Input  dbl_ovrd=off  block_type=slice
      settings: block_version=9.1.01
  Slice1 : xbsIndex_r4/Slice  nbits=0  boolean_output=off  mode=Two Bit Locations  bit1=0  base1=MSB of Input  bit0=18  base0=LSB of Input  dbl_ovrd=off  block_type=slice
      settings: block_version=9.1.01
  delay2 : xbsIndex_r4/Delay  en=off  latency=4  dbl_ovrd=off  reg_retiming=off  block_type=delay
  delay_bram : Subsystem
  dsp48e_mult : Subsystem
  sync_delay_z^-1024 : Subsystem
  dout : Outport
  sync_out : Outport  Port=2
  coeff_out : Outport  Port=3
  taps_out : Outport  Port=4
  wires:
  tap_in/1 -> dsp48e_mult/3(tap_in)
  Reinterpret1/1 -> delay2/1
  delay2/1 -> dsp48e_mult/1(a)
  Reinterpret/1 -> dsp48e_mult/2(b)
  Slice/1 -> Reinterpret/1
  Slice1/1 -> coeff_out/1
  coeff/1 -> Slice1/1, Slice/1
  sync_delay_z^-1024/1(Out1) -> sync_out/1
  sync/1 -> sync_delay_z^-1024/1(In1)
  dsp48e_mult/1(p) -> taps_out/1
  din/1 -> Reinterpret1/1, delay_bram/1(In1)
  delay_bram/1(Out1) -> dout/1

== system pfb_fir_real_plan/filter_01/tap6 ==
  din : Inport
  sync : Inport  Port=2
  coeff : Inport  Port=3
  tap_in : Inport  Port=4
  Delay : xbsIndex_r4/Delay  en=off  latency=8  dbl_ovrd=off  reg_retiming=off  block_type=delay
      settings: xl_area=[0, 0, 0, 0, 0, 0, 0]  block_version=9.1.01
  Delay2 : xbsIndex_r4/Delay  en=off  latency=5  dbl_ovrd=off  reg_retiming=off  block_type=delay
      settings: xl_area=[0, 0, 0, 0, 0, 0, 0]  block_version=9.1.01
  Reinterpret : xbsIndex_r4/Reinterpret  force_arith_type=on  arith_type="Signed  (2's comp)"  force_bin_pt=on  bin_pt=17  block_type=reinterpret
      settings: infoedit="Changes signal type without altering the binary representation.   You can changed the signal between signed and unsigned, and relocate the binary point.<br><br>Hardware notes: In hardware this block costs nothing.<br><br>Example:  Suppose the input is 6 bits wide, signed, with 2 fractional bits, and the output is forced to unsigned with 0 fractional bits.  Then an input of -2.0 (1110.00 in binary 2's complement) becomes an output of 56 (111000 in binary)."  block_version=9.1.01
  Reinterpret1 : xbsIndex_r4/Reinterpret  force_arith_type=on  arith_type="Signed  (2's comp)"  force_bin_pt=on  bin_pt=17  block_type=reinterpret
      settings: infoedit="Changes signal type without altering the binary representation.   You can changed the signal between signed and unsigned, and relocate the binary point.<br><br>Hardware notes: In hardware this block costs nothing.<br><br>Example:  Suppose the input is 6 bits wide, signed, with 2 fractional bits, and the output is forced to unsigned with 0 fractional bits.  Then an input of -2.0 (1110.00 in binary 2's complement) becomes an output of 56 (111000 in binary)."  block_version=9.1.01
  dsp48e_mult : Subsystem
  sync_out : Outport
  tap_out : Outport  Port=2
  wires:
  Delay/1 -> sync_out/1
  din/1 -> Reinterpret1/1
  sync/1 -> Delay/1
  coeff/1 -> Reinterpret/1
  dsp48e_mult/1(p) -> tap_out/1
  Reinterpret1/1 -> Delay2/1
  Delay2/1 -> dsp48e_mult/1(a)
  Reinterpret/1 -> dsp48e_mult/2(b)
  tap_in/1 -> dsp48e_mult/3(tap_in)

== system pfb_fir_real_plan/filter_16/tap1 ==
  din : Inport
  sync : Inport  Port=2
  coeff : Inport  Port=3
  Reinterpret : xbsIndex_r4/Reinterpret  force_arith_type=on  arith_type="Signed  (2's comp)"  force_bin_pt=on  bin_pt=17  block_type=reinterpret
      settings: infoedit="Changes signal type without altering the binary representation.   You can changed the signal between signed and unsigned, and relocate the binary point.<br><br>Hardware notes: In hardware this block costs nothing.<br><br>Example:  Suppose the input is 6 bits wide, signed, with 2 fractional bits, and the output is forced to unsigned with 0 fractional bits.  Then an input of -2.0 (1110.00 in binary 2's complement) becomes an output of 56 (111000 in binary)."  block_version=9.1.01
  Reinterpret1 : xbsIndex_r4/Reinterpret  force_arith_type=on  arith_type="Signed  (2's comp)"  force_bin_pt=on  bin_pt=17  block_type=reinterpret
      settings: infoedit="Changes signal type without altering the binary representation.   You can changed the signal between signed and unsigned, and relocate the binary point.<br><br>Hardware notes: In hardware this block costs nothing.<br><br>Example:  Suppose the input is 6 bits wide, signed, with 2 fractional bits, and the output is forced to unsigned with 0 fractional bits.  Then an input of -2.0 (1110.00 in binary 2's complement) becomes an output of 56 (111000 in binary)."  block_version=9.1.01
  Slice : xbsIndex_r4/Slice  nbits=18  boolean_output=off  mode=Lower Bit Location + Width  bit1=0  base1=MSB of Input  bit0=0  base0=LSB of Input  dbl_ovrd=off  block_type=slice
      settings: block_version=9.1.01
  Slice1 : xbsIndex_r4/Slice  nbits=0  boolean_output=off  mode=Two Bit Locations  bit1=0  base1=MSB of Input  bit0=18  base0=LSB of Input  dbl_ovrd=off  block_type=slice
      settings: block_version=9.1.01
  delay_bram : Subsystem
  dsp48e_mult : Subsystem
  sync_delay_z^-1024 : Subsystem
  dout : Outport
  sync_out : Outport  Port=2
  coeff_out : Outport  Port=3
  taps_out : Outport  Port=4
  wires:
  delay_bram/1(Out1) -> dout/1
  din/1 -> delay_bram/1(In1), Reinterpret1/1
  dsp48e_mult/1(p) -> taps_out/1
  sync/1 -> sync_delay_z^-1024/1(In1)
  sync_delay_z^-1024/1(Out1) -> sync_out/1
  coeff/1 -> Slice/1, Slice1/1
  Slice1/1 -> coeff_out/1
  Slice/1 -> Reinterpret/1
  Reinterpret/1 -> dsp48e_mult/2(b)
  Reinterpret1/1 -> dsp48e_mult/1(a)

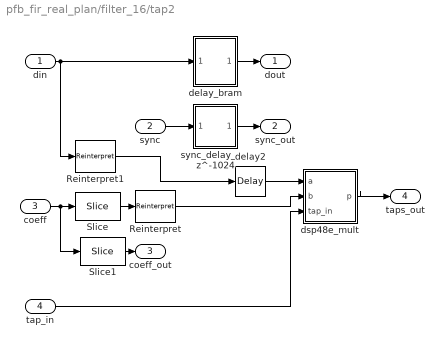
== system pfb_fir_real_plan/filter_16/tap2 ==
  din : Inport
  sync : Inport  Port=2
  coeff : Inport  Port=3
  tap_in : Inport  Port=4
  Reinterpret : xbsIndex_r4/Reinterpret  force_arith_type=on  arith_type="Signed  (2's comp)"  force_bin_pt=on  bin_pt=17  block_type=reinterpret
      settings: infoedit="Changes signal type without altering the binary representation.   You can changed the signal between signed and unsigned, and relocate the binary point.<br><br>Hardware notes: In hardware this block costs nothing.<br><br>Example:  Suppose the input is 6 bits wide, signed, with 2 fractional bits, and the output is forced to unsigned with 0 fractional bits.  Then an input of -2.0 (1110.00 in binary 2's complement) becomes an output of 56 (111000 in binary)."  block_version=9.1.01
  Reinterpret1 : xbsIndex_r4/Reinterpret  force_arith_type=on  arith_type="Signed  (2's comp)"  force_bin_pt=on  bin_pt=17  block_type=reinterpret
      settings: infoedit="Changes signal type without altering the binary representation.   You can changed the signal between signed and unsigned, and relocate the binary point.<br><br>Hardware notes: In hardware this block costs nothing.<br><br>Example:  Suppose the input is 6 bits wide, signed, with 2 fractional bits, and the output is forced to unsigned with 0 fractional bits.  Then an input of -2.0 (1110.00 in binary 2's complement) becomes an output of 56 (111000 in binary)."  block_version=9.1.01
  Slice : xbsIndex_r4/Slice  nbits=18  boolean_output=off  mode=Lower Bit Location + Width  bit1=0  base1=MSB of Input  bit0=0  base0=LSB of Input  dbl_ovrd=off  block_type=slice
      settings: block_version=9.1.01
  Slice1 : xbsIndex_r4/Slice  nbits=0  boolean_output=off  mode=Two Bit Locations  bit1=0  base1=MSB of Input  bit0=18  base0=LSB of Input  dbl_ovrd=off  block_type=slice
      settings: block_version=9.1.01
  delay2 : xbsIndex_r4/Delay  en=off  latency=1  dbl_ovrd=off  reg_retiming=off  block_type=delay
  delay_bram : Subsystem
  dsp48e_mult : Subsystem
  sync_delay_z^-1024 : Subsystem
  dout : Outport
  sync_out : Outport  Port=2
  coeff_out : Outport  Port=3
  taps_out : Outport  Port=4
  wires:
  tap_in/1 -> dsp48e_mult/3(tap_in)
  Reinterpret1/1 -> delay2/1
  delay2/1 -> dsp48e_mult/1(a)
  Reinterpret/1 -> dsp48e_mult/2(b)
  Slice/1 -> Reinterpret/1
  Slice1/1 -> coeff_out/1
  coeff/1 -> Slice1/1, Slice/1
  sync_delay_z^-1024/1(Out1) -> sync_out/1
  sync/1 -> sync_delay_z^-1024/1(In1)
  dsp48e_mult/1(p) -> taps_out/1
  din/1 -> Reinterpret1/1, delay_bram/1(In1)
  delay_bram/1(Out1) -> dout/1

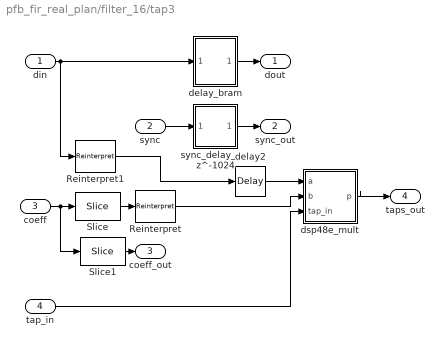
== system pfb_fir_real_plan/filter_16/tap3 ==
  din : Inport
  sync : Inport  Port=2
  coeff : Inport  Port=3
  tap_in : Inport  Port=4
  Reinterpret : xbsIndex_r4/Reinterpret  force_arith_type=on  arith_type="Signed  (2's comp)"  force_bin_pt=on  bin_pt=17  block_type=reinterpret
      settings: infoedit="Changes signal type without altering the binary representation.   You can changed the signal between signed and unsigned, and relocate the binary point.<br><br>Hardware notes: In hardware this block costs nothing.<br><br>Example:  Suppose the input is 6 bits wide, signed, with 2 fractional bits, and the output is forced to unsigned with 0 fractional bits.  Then an input of -2.0 (1110.00 in binary 2's complement) becomes an output of 56 (111000 in binary)."  block_version=9.1.01
  Reinterpret1 : xbsIndex_r4/Reinterpret  force_arith_type=on  arith_type="Signed  (2's comp)"  force_bin_pt=on  bin_pt=17  block_type=reinterpret
      settings: infoedit="Changes signal type without altering the binary representation.   You can changed the signal between signed and unsigned, and relocate the binary point.<br><br>Hardware notes: In hardware this block costs nothing.<br><br>Example:  Suppose the input is 6 bits wide, signed, with 2 fractional bits, and the output is forced to unsigned with 0 fractional bits.  Then an input of -2.0 (1110.00 in binary 2's complement) becomes an output of 56 (111000 in binary)."  block_version=9.1.01
  Slice : xbsIndex_r4/Slice  nbits=18  boolean_output=off  mode=Lower Bit Location + Width  bit1=0  base1=MSB of Input  bit0=0  base0=LSB of Input  dbl_ovrd=off  block_type=slice
      settings: block_version=9.1.01
  Slice1 : xbsIndex_r4/Slice  nbits=0  boolean_output=off  mode=Two Bit Locations  bit1=0  base1=MSB of Input  bit0=18  base0=LSB of Input  dbl_ovrd=off  block_type=slice
      settings: block_version=9.1.01
  delay2 : xbsIndex_r4/Delay  en=off  latency=2  dbl_ovrd=off  reg_retiming=off  block_type=delay
  delay_bram : Subsystem
  dsp48e_mult : Subsystem
  sync_delay_z^-1024 : Subsystem
  dout : Outport
  sync_out : Outport  Port=2
  coeff_out : Outport  Port=3
  taps_out : Outport  Port=4
  wires:
  delay_bram/1(Out1) -> dout/1
  din/1 -> delay_bram/1(In1), Reinterpret1/1
  dsp48e_mult/1(p) -> taps_out/1
  sync/1 -> sync_delay_z^-1024/1(In1)
  sync_delay_z^-1024/1(Out1) -> sync_out/1
  coeff/1 -> Slice/1, Slice1/1
  Slice1/1 -> coeff_out/1
  Slice/1 -> Reinterpret/1
  Reinterpret/1 -> dsp48e_mult/2(b)
  delay2/1 -> dsp48e_mult/1(a)
  Reinterpret1/1 -> delay2/1
  tap_in/1 -> dsp48e_mult/3(tap_in)
